simulink library "driver_interface_lib"  (R2022b)
settings: Solver=VariableStepAuto  StartTime=0.0  StopTime=10.0  RelTol=1e-3
undefined symbols (not defined in the file): MI_STATUSES
libraries: $bdroot x3, simulink x1
settings Model: Creator=dr_pa  LastModifiedBy=LinF

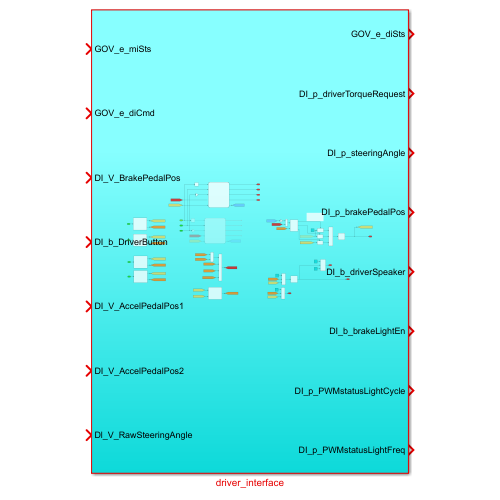
[thumbnail: Simulink's stored preview of the top-level diagram]
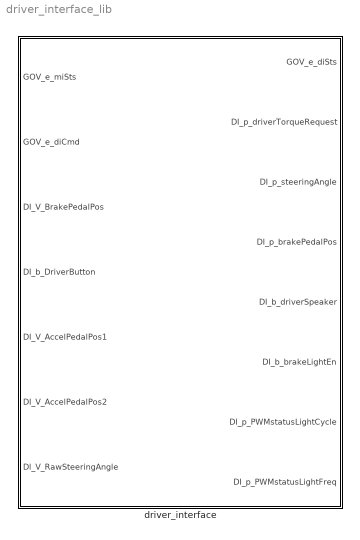
== system driver_interface_lib ==
  driver_interface : Subsystem

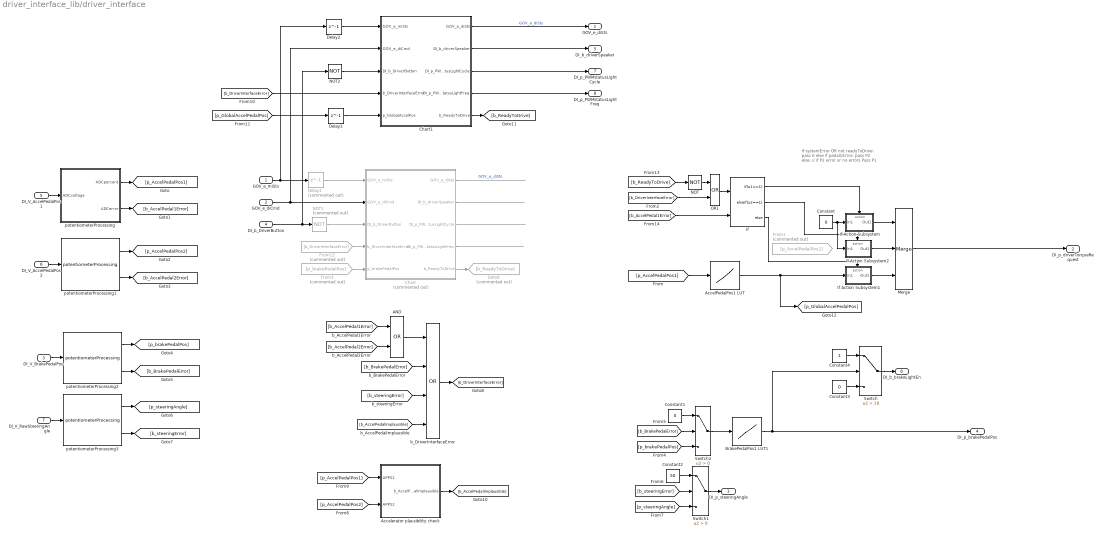
== system driver_interface_lib/driver_interface ==
  note: if systemError OR not readyToDrive:
      | 	pass 0
      | else if pedal1Error:
      | 	pass P2
      | else: // if P2 error or no errors
      | 	Pass P1
  GOV_e_miSts : Inport
  GOV_e_diCmd : Inport  Port=2
  DI_V_BrakePedalPos : Inport  Port=3
  DI_b_DriverButton : Inport  Port=4
  DI_V_AccelPedalPos1 : Inport  Port=5
  DI_V_AccelPedalPos2 : Inport  Port=6
  Dl_V_RawSteeringAngle : Inport  Port=7
  AND : Logic  Operator=OR  AllPortsSameDT=off  OutDataTypeStr=boolean
  AccelPedalPos1 LUT : Lookup_n-D  NumberOfTableDimensions=1  BreakpointsForDimension1=[0 1 2 3 4 5 6 7 8 9 10 11 12 13 14 15 16 17 18 19 20 21 22 23 24 25 26 27 28 29 30 31 32 33 34 35 36 37 38 39 40 41 42 43 44 45 46 47 48 49 50 51 52 53 54 55 56 57 58 59 60 61 62 63 64 65 66 67 68 69 70 71 72 73 74 75 76 77 78 79 80 81 82 83 84 85 86 87 88 89 90 91 92 93 94 95 96 97 98 99]  Table=[0 0 0 0 0 0 0 0 0 0 0 0 0 0 0 0 0 0 0 0 0 0 1.85185185185185 3.7037037037037 5.55555555555556 7.40740740740741 9.25925925925926 11.1111111111111 12.962962962963 14.8148148148148 16.6666666666667 18.5185185185185 20.3703703703704 22.2222222222222 24.0740740740741 25.9259259259259 27.7777777777778 29.6296296296296 31.4814814814815 33.3333333333333 35.1851851851852 37.037037037037 38.8888888888889 40.7407407407407 42.5925925925926 44.4444444444444 46.2962962962963 48.1481481481481 50 51.8518518518519 53.7037037037037 55.5555555555556 57.4074074074074 59.2592592592593 61.1111111111111 62.962962962963 64.8148148148148 66.6666666666667 68.5185185185185 70.3703703703704 72.2222222222222 74.0740740740741 75.9259259259259 77.7777777777778 79.6296296296296 81.4814814814815 83.3333333333333 85.1851851851852 87.037037037037 88.8888888888889 90.7407407407407 92.5925925925926 94.4444444444444 96.2962962962963 98.1481481481482 100 100 100 100 100 100 100 100 100 100 100 100 100 100 100 100 100 100 100 100 100 100 100 100 100]  ExtrapMethod=Clip  InternalRulePriority=Speed  RndMeth=Simplest
  Accelerator plausibility check : Subsystem
  BrakePedalPos1 LUT1 : Lookup_n-D  NumberOfTableDimensions=1  BreakpointsForDimension1=[0 5 10 15 20 25 30 35 40 45 50 55 60 65 70 75 80 85 90 95 100]  Table=[0 5 10 15 20 25 30 35 40 45 50 55 60 65 70 75 80 85 90 95 100]  ExtrapMethod=Clip  InternalRulePriority=Speed  RndMeth=Simplest
  Chart : Stateflow chart  Commented=on  TreatAsAtomicUnit=on
  Chart1 : Stateflow chart  TreatAsAtomicUnit=on
  Constant : Constant  Value=0  OutDataTypeStr=single
  Constant1 : Constant  Value=0  OutDataTypeStr=single
  Constant2 : Constant  Value=50  OutDataTypeStr=single
  Constant3 : Constant  Value=0  OutDataTypeStr=single
  Constant4 : Constant  OutDataTypeStr=single
  Delay1 : Delay  Commented=on  DelayLength=1  InitialCondition=MI_STATUSES.UNKNOWN
  Delay2 : Delay  DelayLength=1  InitialCondition=MI_STATUSES.UNKNOWN
  Delay3 : Delay  DelayLength=1  InitialCondition=0
  From1 : From  Commented=on  GotoTag=p_AccelPedalPos2
  From12 : From  Commented=on  GotoTag=b_DriverInterfaceError
  From3 : From  Commented=on  GotoTag=p_brakePedalPos
  Goto9 : Goto  Commented=on  GotoTag=b_ReadyToDrive
  If : If  NumInputs=2  IfExpression=u1==1  ElseIfExpressions=u2==1
  If Action Subsystem : Subsystem  TreatAsAtomicUnit=on
  If Action Subsystem1 : Subsystem  TreatAsAtomicUnit=on
  If Action Subsystem2 : Subsystem  TreatAsAtomicUnit=on
  Merge : Merge  Inputs=3
  NOT : Logic  Operator=NOT  IconShape=distinctive  AllPortsSameDT=off  OutDataTypeStr=boolean
  NOT1 : Logic  Commented=on  Operator=NOT  IconShape=distinctive  AllPortsSameDT=off  OutDataTypeStr=boolean
  NOT2 : Logic  Operator=NOT  IconShape=distinctive  AllPortsSameDT=off  OutDataTypeStr=boolean
  OR1 : Logic  Operator=OR  AllPortsSameDT=off  OutDataTypeStr=boolean
  Switch : Switch  Criteria=u2 > Threshold  Threshold=10  SaturateOnIntegerOverflow=off  InputSameDT=off
  Switch1 : Switch  Criteria=u2 > Threshold  SaturateOnIntegerOverflow=off  InputSameDT=off
  Switch2 : Switch  Criteria=u2 > Threshold  SaturateOnIntegerOverflow=off  InputSameDT=off
  b_DriverInterfaceError : Logic  Operator=OR  Inputs=4  AllPortsSameDT=off  OutDataTypeStr=boolean
  potentiometerProcessing : Subsystem
  potentiometerProcessing1 : $bdroot/driver_interface/potentiometerProcessing  SystemSampleTime=-1  VariantActivationTime=update diagram  Latency=0  AutoFrameSizeCalculation=off
  potentiometerProcessing2 : $bdroot/driver_interface/potentiometerProcessing  SystemSampleTime=-1  VariantActivationTime=update diagram  Latency=0  AutoFrameSizeCalculation=off
  potentiometerProcessing3 : $bdroot/driver_interface/potentiometerProcessing  SystemSampleTime=-1  VariantActivationTime=update diagram  Latency=0  AutoFrameSizeCalculation=off
  GOV_e_diSts : Outport
  DI_p_driverTorqueRequest : Outport  Port=2
  DI_p_steeringAngle : Outport  Port=3
  DI_p_brakePedalPos : Outport  Port=4
  DI_b_driverSpeaker : Outport  Port=5
  DI_b_brakeLightEn : Outport  Port=6
  DI_p_PWMstatusLightCycle : Outport  Port=7
  DI_p_PWMstatusLightFreq : Outport  Port=8
  wires:
  [b_AccelPedalImplausible] -> b_DriverInterfaceError/4
  Accelerator plausibility check/1(b_AccelPedalImplausible) -> [b_AccelPedalImplausible]
  [p_AccelPedalPos2] -> Accelerator plausibility check/2(APPS2)
  [p_AccelPedalPos1] -> Accelerator plausibility check/1(APPS1)
  Chart/4(DI_p_PWMstatusLightFreq) -> ?
  Chart/3(DI_p_PWMstatusLightCycle) -> ?
  Constant4/1 -> Switch/1
  Constant3/1 -> Switch/3
  Switch/1 -> DI_b_brakeLightEn/1
  Chart/1(GOV_e_diSts) -> ?  "GOV_e_diSts"
  Merge/1 -> DI_p_driverTorqueRequest/1
  DI_V_AccelPedalPos1/1 -> potentiometerProcessing/1(ADCvoltage)
  potentiometerProcessing/1(ADCpercent) -> [p_AccelPedalPos1]
  potentiometerProcessing/2(ADCerror) -> [b_AccelPedal1Error]
  potentiometerProcessing1/1 -> [p_AccelPedalPos2]
  potentiometerProcessing1/2 -> [b_AccelPedal2Error]
  potentiometerProcessing2/2 -> [b_BrakePedalError]
  potentiometerProcessing2/1 -> [p_brakePedalPos]
  potentiometerProcessing3/1 -> [p_steeringAngle]
  potentiometerProcessing3/2 -> [b_steeringError]
  If Action Subsystem/1(Out1) -> Merge/1
  If/1 -> If Action Subsystem/Action
  If Action Subsystem1/1(Out1) -> Merge/3
  [p_AccelPedalPos1] -> AccelPedalPos1 LUT/1
  [b_AccelPedal1Error] -> If/2
  [b_BrakePedalError] -> Switch2/2
  Constant1/1 -> Switch2/1
  [p_brakePedalPos] -> Switch2/3
  Switch2/1 -> BrakePedalPos1 LUT1/1
  Constant2/1 -> Switch1/1
  Switch1/1 -> DI_p_steeringAngle/1
  [b_steeringError] -> Switch1/2
  [p_steeringAngle] -> Switch1/3
  [b_AccelPedal2Error] -> AND/2
  [b_AccelPedal1Error] -> AND/1
  AND/1 -> b_DriverInterfaceError/1
  [b_BrakePedalError] -> b_DriverInterfaceError/2
  [b_steeringError] -> b_DriverInterfaceError/3
  From12/1 -> Chart/4(b_DriverInterfaceError)
  Chart/2(DI_b_driverSpeaker) -> ?
  Constant/1 -> If Action Subsystem2/1(In1), If Action Subsystem/1(In1)
  If/2 -> If Action Subsystem2/Action
  If/3 -> If Action Subsystem1/Action
  Chart/5(b_ReadyToDrive) -> Goto9/1
  OR1/1 -> If/1
  [b_DriverInterfaceError] -> OR1/2
  [b_ReadyToDrive] -> NOT/1
  NOT/1 -> OR1/1
  b_DriverInterfaceError/1 -> [b_DriverInterfaceError]
  DI_V_AccelPedalPos2/1 -> potentiometerProcessing1/1
  DI_V_BrakePedalPos/1 -> potentiometerProcessing2/1
  Dl_V_RawSteeringAngle/1 -> potentiometerProcessing3/1
  From3/1 -> Chart/5(p_brakePedalPos)
  BrakePedalPos1 LUT1/1 -> DI_p_brakePedalPos/1, Switch/2
  Delay1/1 -> Chart/1(GOV_e_miSts)
  NOT1/1 -> Chart/3(DI_b_DriverButton)
  Chart1/4(DI_p_PWMstatusLightFreq) -> DI_p_PWMstatusLightFreq/1
  Delay2/1 -> Chart1/1(GOV_e_miSts)
  NOT2/1 -> Chart1/3(DI_b_DriverButton)
  GOV_e_diCmd/1 -> Chart/2(GOV_e_diCmd), Chart1/2(GOV_e_diCmd)
  DI_b_DriverButton/1 -> NOT1/1, NOT2/1
  [p_GlobalAccelPedalPos] -> Delay3/1
  Chart1/2(DI_b_driverSpeaker) -> DI_b_driverSpeaker/1
  Chart1/5(b_ReadyToDrive) -> [b_ReadyToDrive]
  Chart1/3(DI_p_PWMstatusLightCycle) -> DI_p_PWMstatusLightCycle/1
  GOV_e_miSts/1 -> Delay1/1, Delay2/1
  [b_DriverInterfaceError] -> Chart1/4(b_DriverInterfaceError)
  Chart1/1(GOV_e_diSts) -> GOV_e_diSts/1  "GOV_e_diSts"
  If Action Subsystem2/1(Out1) -> Merge/2
  Delay3/1 -> Chart1/5(p_GlobalAccelPos)
  AccelPedalPos1 LUT/1 -> [p_GlobalAccelPedalPos], If Action Subsystem1/1(In1)

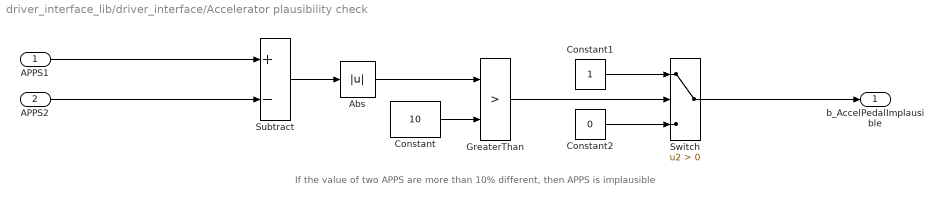
== system driver_interface_lib/driver_interface/Accelerator plausibility check ==
  note: If the value of two APPS are more than 10% different, then APPS is implausible
  APPS1 : Inport
  APPS2 : Inport  Port=2
  Abs : Abs  SaturateOnIntegerOverflow=off
  Constant : Constant  Value=10
  Constant1 : Constant
  Constant2 : Constant  Value=0
  GreaterThan : RelationalOperator  Operator=>  OutDataTypeStr=boolean  RndMeth=Simplest  InputSameDT=off
  Subtract : Sum  Inputs=+-
  Switch : Switch  Criteria=u2 > Threshold  SaturateOnIntegerOverflow=off  InputSameDT=off
  b_AccelPedalImplausible : Outport
  wires:
  Switch/1 -> b_AccelPedalImplausible/1
  Constant2/1 -> Switch/3
  Constant1/1 -> Switch/1
  GreaterThan/1 -> Switch/2
  Constant/1 -> GreaterThan/2
  Abs/1 -> GreaterThan/1
  Subtract/1 -> Abs/1
  APPS2/1 -> Subtract/2
  APPS1/1 -> Subtract/1

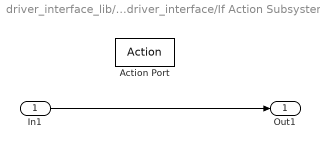
== system driver_interface_lib/driver_interface/If Action Subsystem ==
  In1 : Inport
  Action Port : ActionPort
  Out1 : Outport
  wires:
  In1/1 -> Out1/1

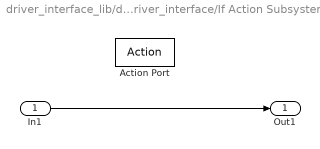
== system driver_interface_lib/driver_interface/If Action Subsystem1 ==
  In1 : Inport
  Action Port : ActionPort
  Out1 : Outport
  wires:
  In1/1 -> Out1/1

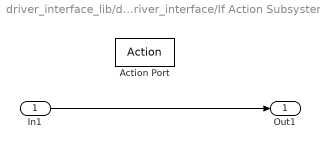
== system driver_interface_lib/driver_interface/If Action Subsystem2 ==
  In1 : Inport
  Action Port : ActionPort
  Out1 : Outport
  wires:
  In1/1 -> Out1/1

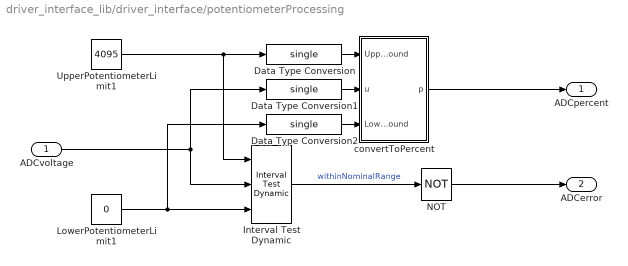
== system driver_interface_lib/driver_interface/potentiometerProcessing ==
  ADCvoltage : Inport
  Data Type Conversion : DataTypeConversion  OutDataTypeStr=single  SaturateOnIntegerOverflow=off  RndMeth=Floor
  Data Type Conversion1 : DataTypeConversion  OutDataTypeStr=single  SaturateOnIntegerOverflow=off  RndMeth=Floor
  Data Type Conversion2 : DataTypeConversion  OutDataTypeStr=single  SaturateOnIntegerOverflow=off  RndMeth=Floor
  Interval Test Dynamic : simulink/Logic and Bit Operations/Interval Test Dynamic  IntervalClosedRight=on  IntervalClosedLeft=on  OutDataTypeStr=boolean
  LowerPotentiometerLimit1 : Constant  Value=0  OutDataTypeStr=double
  NOT : Logic  Operator=NOT  IconShape=distinctive  AllPortsSameDT=off  OutDataTypeStr=boolean
  UpperPotentiometerLimit1 : Constant  Value=4095  OutDataTypeStr=double
  convertToPercent : Subsystem
  ADCpercent : Outport
  ADCerror : Outport  Port=2
  wires:
  LowerPotentiometerLimit1/1 -> Interval Test Dynamic/3, Data Type Conversion2/1
  UpperPotentiometerLimit1/1 -> Interval Test Dynamic/1, Data Type Conversion/1
  Interval Test Dynamic/1 -> NOT/1  "withinNominalRange"
  convertToPercent/1(p) -> ADCpercent/1
  ADCvoltage/1 -> Interval Test Dynamic/2, Data Type Conversion1/1
  NOT/1 -> ADCerror/1
  Data Type Conversion/1 -> convertToPercent/1(UpperBound)
  Data Type Conversion1/1 -> convertToPercent/2(u)
  Data Type Conversion2/1 -> convertToPercent/3(LowerBound)

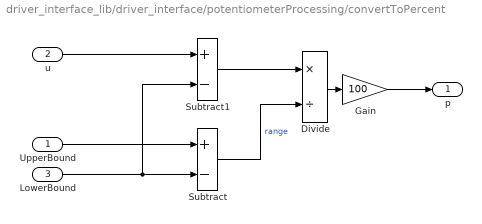
== system driver_interface_lib/driver_interface/potentiometerProcessing/convertToPercent ==
  UpperBound : Inport
  u : Inport  Port=2
  LowerBound : Inport  Port=3
  Divide : Product  Inputs=*/
  Gain : Gain  Gain=100
  Subtract : Sum  Inputs=+-
  Subtract1 : Sum  Inputs=+-
  p : Outport
  wires:
  Divide/1 -> Gain/1
  Subtract/1 -> Divide/2  "range"
  UpperBound/1 -> Subtract/1
  Gain/1 -> p/1
  Subtract1/1 -> Divide/1
  u/1 -> Subtract1/1
  LowerBound/1 -> Subtract1/2, Subtract/2

== stateflow chart driver_interface_lib/driver_interface/Chart1 ==
  state INIT
    en:
    GOV_e_diSts = DI_STATUSES.DI_STS_INIT;
    b_ReadyToDrive=false;
    DI_b_driverSpeaker = false;
    DI_p_PWMstatusLightCycle = 0;
    DI_p_PWMstatusLightFreq = 1;
  state DI_running
    state Waiting_for_driver
      en:
      GOV_e_diSts = ...
      DI_STATUSES.WAITING_FOR_DRVR;
      DI_p_PWMstatusLightCycle = 50;
      DI_p_PWMstatusLightFreq = 1;
    state Driver_requested_start
      en:
      GOV_e_diSts = DI_STATUSES.DRV_START_REQ;
      DI_p_PWMstatusLightCycle = 50;
      DI_p_PWMstatusLightFreq = 10;
    state Motor_ready
      en:
      DI_p_PWMstatusLightCycle = 100;
      DI_p_PWMstatusLightFreq = 10;
    state Ready_to_drive
      en:
      b_ReadyToDrive = true;
      GOV_e_diSts = DI_RUNNING;
      DI_p_PWMstatusLightCycle = 100; %Always on
      DI_p_PWMstatusLightFreq = 10;
      state SpeakerOn_
        en:
        DI_b_driverSpeaker = true;
      state SpeakerOff
        en:
        DI_b_driverSpeaker = false;
      (default) -> SpeakerOn_
      SpeakerOn_ -> SpeakerOff : after(2,sec)
    Waiting_for_driver -> Driver_requested_start : [(DI_b_DriverButton==1)]
    Driver_requested_start -> Motor_ready : [GOV_e_miSts == MI_STATUSES.READY]
    Motor_ready -> Ready_to_drive : [GOV_e_diCmd ==...
        |  DI_CMD.READY_TO_DRIVE  && (p_GlobalAccelPos == 0)]
  state DI_error
    en:
    GOV_e_diSts = DI_STATUSES.DI_ERROR;
  state Vehicle_coasting
    en:
    b_ReadyToDrive = false;
    GOV_e_diSts = DI_STATUSES.DI_IDLE;
  (default) -> INIT
  Ready_to_drive -> INIT [order 2] : [GOV_e_miSts == MI_STATUSES.OFF]
  INIT -> Waiting_for_driver : after(10,sec)
  DI_running -> DI_error : [b_DriverInterfaceError==1]
  Ready_to_drive -> Vehicle_coasting [order 1] : [GOV_e_diCmd ==...
      |  DI_CMD.SYSTEM_ERROR]
  data: GOV_e_miSts input Enum: MI_STATUSES; GOV_e_diCmd input Enum: DI_CMD; DI_b_DriverButton input; GOV_e_diSts output Enum: DI_STATUSES size=1; b_DriverInterfaceError input; DI_b_driverSpeaker output boolean; DI_p_PWMstatusLightCycle output; DI_p_PWMstatusLightFreq output; b_ReadyToDrive output boolean; p_GlobalAccelPos input

== stateflow chart driver_interface_lib/driver_interface/Chart ==
  state INIT
    en:
    GOV_e_diSts = DI_STATUSES.DI_STS_INIT;
    b_ReadyToDrive=false;
    DI_b_driverSpeaker = false;
    DI_p_PWMstatusLightCycle = 0;
    DI_p_PWMstatusLightFreq = 1;
  state DI_running
    state Waiting_for_driver
      en:
      GOV_e_diSts = ...
      DI_STATUSES.WAITING_FOR_DRVR;
      DI_p_PWMstatusLightCycle = 50;
      DI_p_PWMstatusLightFreq = 1;
    state Driver_requested_start
      en:
      GOV_e_diSts = DI_STATUSES.DRV_START_REQ;
      DI_p_PWMstatusLightCycle = 50;
      DI_p_PWMstatusLightFreq = 10;
    state Motor_ready
      en:
      DI_p_PWMstatusLightCycle = 100;
      DI_p_PWMstatusLightFreq = 10;
    state Ready_to_drive
      en:
      b_ReadyToDrive = true;
      GOV_e_diSts = DI_RUNNING;
      DI_p_PWMstatusLightCycle = 100; %Always on
      DI_p_PWMstatusLightFreq = 10;
      state SpeakerOn_
        en:
        DI_b_driverSpeaker = true;
      state SpeakerOff
        en:
        DI_b_driverSpeaker = false;
      (default) -> SpeakerOn_
      SpeakerOn_ -> SpeakerOff : after(2,sec)
    Waiting_for_driver -> Driver_requested_start : [(DI_b_DriverButton==1)]
    Driver_requested_start -> Motor_ready : [GOV_e_miSts == MI_STATUSES.READY]
    Motor_ready -> Ready_to_drive : [GOV_e_diCmd ==...
        |  DI_CMD.READY_TO_DRIVE  && (p_brakePedalPos>10)]
  state DI_error
    en:
    GOV_e_diSts = DI_STATUSES.DI_ERROR;
  state Vehicle_coasting
    en:
    b_ReadyToDrive = false;
    GOV_e_diSts = DI_STATUSES.DI_IDLE;
  (default) -> INIT
  Ready_to_drive -> INIT [order 2] : [GOV_e_miSts == MI_STATUSES.OFF]
  INIT -> Waiting_for_driver : after(10,sec)
  DI_running -> DI_error : [b_DriverInterfaceError==1]
  Ready_to_drive -> Vehicle_coasting [order 1] : [GOV_e_diCmd ==...
      |  DI_CMD.SYSTEM_ERROR]
  data: GOV_e_miSts input Enum: MI_STATUSES; GOV_e_diCmd input Enum: DI_CMD; DI_b_DriverButton input; GOV_e_diSts output Enum: DI_STATUSES size=1; b_DriverInterfaceError input; DI_b_driverSpeaker output boolean; DI_p_PWMstatusLightCycle output; DI_p_PWMstatusLightFreq output; b_ReadyToDrive output boolean; p_brakePedalPos input
